simulink subsystem "StateSpaceControllerRobust_SubSystem"  (R2020b)
settings: Solver=VariableStepAuto  StartTime=0.0  StopTime=10.0  RelTol=1e-3
undefined symbols (not defined in the file): DiscIntNeverNeededParam, drv, enable_Robust_Controller, K, Ki, Nu, Nx, Ts
settings Model: Creator=umberto  LastModifiedBy=Musta

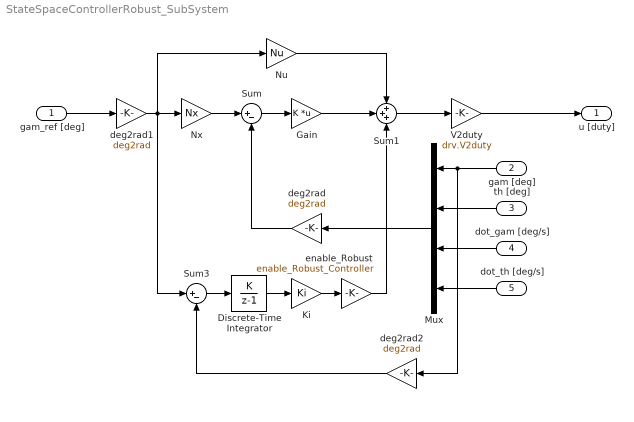
== system StateSpaceControllerRobust_SubSystem ==
  gam_ref [deg] : Inport
  gam [deg] : Inport  Port=2
  th [deg] : Inport  Port=3
  dot_gam [deg/s] : Inport  Port=4
  dot_th [deg/s] : Inport  Port=5
  Discrete-Time Integrator : DiscreteIntegrator  IntegratorMethod=Accumulation: Forward Euler  SampleTime=Ts  ICPrevOutput=DiscIntNeverNeededParam  ICPrevScaledInput=DiscIntNeverNeededParam
  Gain : Gain  Gain=K  Multiplication=Matrix(K*u)
  Ki : Gain  Gain=Ki
  Mux : Mux
  Nu : Gain  Gain=Nu
  Nx : Gain  Gain=Nx
  Sum : Sum  Inputs=|+-
  Sum1 : Sum  Inputs=+++
  Sum3 : Sum  Inputs=|+-
  V2duty : Gain  Gain=drv.V2duty
  deg2rad : Gain  Gain=deg2rad
  deg2rad1 : Gain  Gain=deg2rad
  deg2rad2 : Gain  Gain=deg2rad
  enable_Robust : Gain  Gain=enable_Robust_Controller
  u [duty] : Outport
  wires:
  gam [deg]/1 -> Mux/1, deg2rad2/1
  th [deg]/1 -> Mux/2
  dot_gam [deg/s]/1 -> Mux/3
  dot_th [deg/s]/1 -> Mux/4
  Mux/1 -> deg2rad/1
  gam_ref [deg]/1 -> deg2rad1/1
  V2duty/1 -> u [duty]/1
  Sum1/1 -> V2duty/1
  deg2rad/1 -> Sum/2
  Gain/1 -> Sum1/2
  Sum/1 -> Gain/1
  deg2rad1/1 -> Nu/1, Nx/1, Sum3/1
  Nx/1 -> Sum/1
  Nu/1 -> Sum1/1
  deg2rad2/1 -> Sum3/2
  Sum3/1 -> Discrete-Time Integrator/1
  Discrete-Time Integrator/1 -> Ki/1
  enable_Robust/1 -> Sum1/3
  Ki/1 -> enable_Robust/1
